simulink model "Save_30_04_20"  (R2019b)
settings: Solver=FixedStepAuto  StartTime=0.0  StopTime=20  FixedStep=0.0001  RelTol=1e-8  AbsTol=1e-9
values from neighbouring files (symbols this model uses):
  Festar = Fs-L*[1 0]    [TestDIST_EFFECT_DCmotor.m]
  Gestar = [Gs L]    [TestDIST_EFFECT_DCmotor.m]
  KK = dlqr(Fs,Gs,Q,R)    [TestDIST_EFFECT_DCmotor.m]
  Ts = 0.001    [TestDIST_EFFECT_DCmotor.m]
settings Model: Creator=oboe  LastModifiedBy=Luca
settings SolverCC: AutoScaleAbsTol=off
settings DataIOCC: ReturnWorkspaceOutputs=off
settings DebuggingCC: ArithmeticOperatorsInVariantConditions=warning
settings SFSimCC: SimUseLocalCustomCode=off  CustomCodeUndefinedFunction=UseInterfaceOnly
settings RTWCC: RTWUseLocalCustomCode=off
settings CodeAppCC: StateflowObjectComments=on

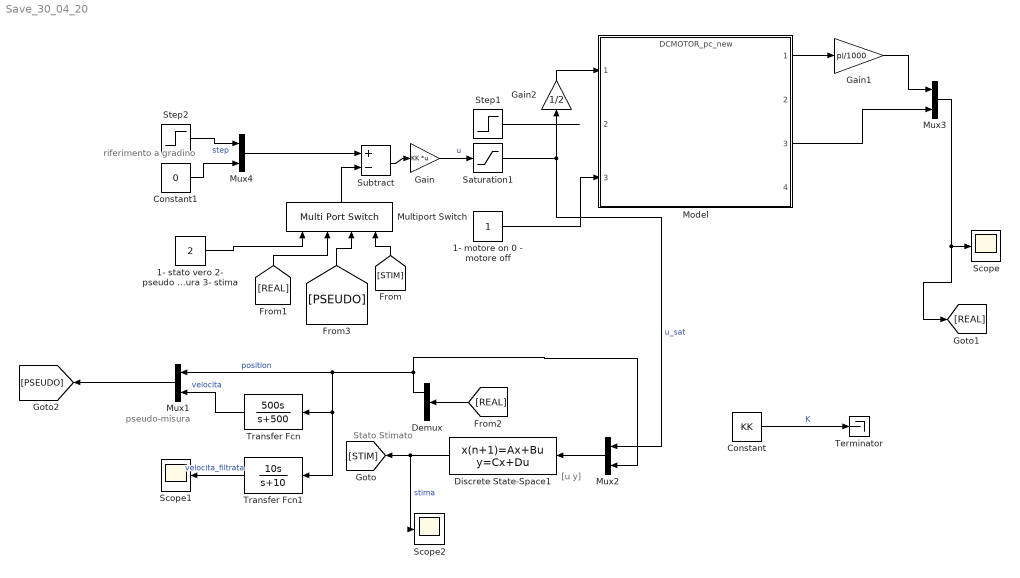
== system Save_30_04_20 ==
  note: pseudo-misura
  note: [u
      | y]
  note: Stato
      | Stimato
  note: riferimento
      | a gradino
  1- motore on 0 - motore off : Constant
  1- stato vero 2- pseudo misura 3- stima : Constant  Value=2
  Constant : Constant  Value=KK
  Constant1 : Constant  Value=0
  Demux : Demux  Outputs=2
  Discrete State-Space1 : DiscreteStateSpace  A=Festar  B=Gestar  C=eye(2)  D=[0 0; 0 0]  InitialCondition=[0 0]'  SampleTime=Ts
  Gain : Gain  Gain=KK  Multiplication=Matrix(K*u)
  Gain1 : Gain  Gain=pi/1000
  Gain2 : Gain  Gain=1/2
  Model : ModelReference  ModelNameDialog=DCMOTOR_pc_new.slxp  ModelReferenceVersion=1.21  CopyOfModelProtected=on
  Multiport Switch : MultiPortSwitch
  Mux{1..4} (4 alike) : Mux  Inputs=2
  Saturation1 : Saturate  UpperLimit=6  LowerLimit=-6
  Scope : Scope
  Scope1 : Scope
  Scope2 : Scope
  Step1 : Step  Time=3  After=.1  SampleTime=0
  Step2 : Step  SampleTime=0
  Subtract : Sum  Inputs=+-
  Terminator : Terminator
  Transfer Fcn : TransferFcn  Numerator=[500 0]  Denominator=[1 500]
  Transfer Fcn1 : TransferFcn  Numerator=[10 0]  Denominator=[1 10]
  wires:
  Mux3/1 -> [REAL], Scope/1
  Subtract/1 -> Gain/1
  Demux/1 -> Mux2/2, Transfer Fcn1/1, Transfer Fcn/1, Mux1/1  "position"
  Transfer Fcn/1 -> Mux1/2  "velocita"
  Mux2/1 -> Discrete State-Space1/1
  Mux1/1 -> [PSEUDO]
  1- stato vero 2- pseudo misura 3- stima/1 -> Multiport Switch/1
  Multiport Switch/1 -> Subtract/2
  Saturation1/1 -> Mux2/1, Gain2/1  "u_sat"
  Step1/1 -> ?
  Gain/1 -> Saturation1/1  "u"
  Discrete State-Space1/1 -> [STIM], Scope2/1  "stima"
  Constant1/1 -> Mux4/2
  Step2/1 -> Mux4/1  "step"
  Mux4/1 -> Subtract/1
  Model/3 -> Mux3/2
  Gain1/1 -> Mux3/1
  Model/1 -> Gain1/1
  1- motore on 0 - motore off/1 -> Model/3
  Gain2/1 -> Model/1
  [STIM] -> Multiport Switch/4
  [REAL] -> Demux/1
  [REAL] -> Multiport Switch/2
  [PSEUDO] -> Multiport Switch/3
  Transfer Fcn1/1 -> Scope1/1  "velocita_filtrata"
  Constant/1 -> Terminator/1  "K"
